simulink model "ComplianceSpeedgoat"  (R2025a)
settings: Solver=FixedStepAuto  StartTime=0.0  StopTime=inf  RelTol=1e-3
undefined symbols (not defined in the file or in its folder): HS, IO291
libraries: slrealtimeethercatlib x11, aru_toolbox x6, speedgoatlib_IO691 x1, speedgoatlib_IO291 x1
settings Model: SimulationMode=external  ExtModeEnableFloating=off  Creator=Blue Fifth  LastModifiedBy=user
settings SolverCC: ConcurrentTasks=on  PositivePriorityOrder=on  AutoInsertRateTranBlk=on
settings OptimizationCC: BlockReduction=off  OptimizeBlockIOStorage=off
settings DebuggingCC: TasksWithSamePriorityMsg=none
settings HardwareCC: ProdBitPerLong=64.0  ProdLongLongMode=on  ProdHWDeviceType=Intel->x86-64 (Linux 64)
settings RTWCC: SystemTargetFile=speedgoat.tlc  TemplateMakefile=slrealtime_default_tmf  Toolchain=Simulink Real-Time Toolchain  BuildConfiguration=Faster Runs  CodeExecutionProfiling=on  TargetLang=C++  GPUComputeCapability=3.5  Description=Speedgoat Real-Time Target Machine
settings SimulinkRealTimeTargetCC: SLRTFileLogMaxRuns=1.0  ExtModeMaxTrigDuration=10.0  ExtModeStaticAllocSize=1000000.0  ExtModeTransport=0.0  MultiwordLength=2048.0  DynamicStringBufferSize=256.0  PreserveMATLABNamespacesInGeneratedCode=on  SubcomponentCodeInterfacePackaging=Reusable function  InstructionSetFMA=off  LogToMDFFile=off

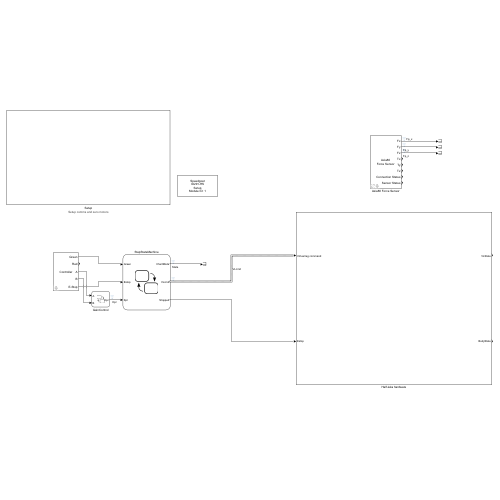
[thumbnail: Simulink's stored preview of the top-level diagram]
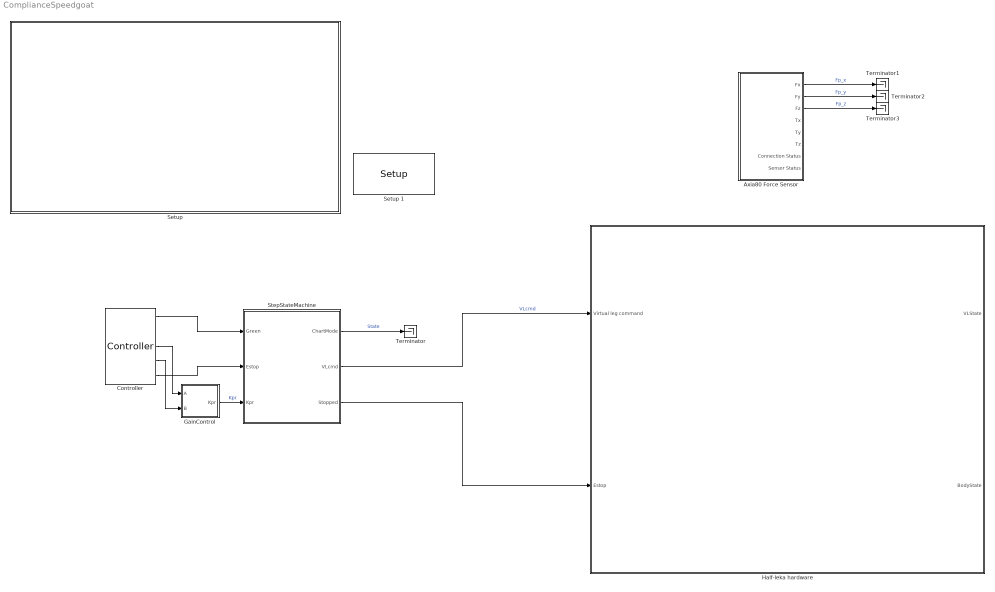
== system ComplianceSpeedgoat ==
  Axia80 Force Sensor : Subsystem  AncestorBlock=aru_toolbox/Axia80 Force Sensor  mask(Axia80 Force Sensor){resetBias=on, calibrationRangeParam=Range 0 (500N Fxy, 900N Fz, 20Nm Txyz), calibrationRangeTable={'0','500N','900N','20Nm'; '1','200N','360N','8Nm'}, sampleRateParam=975Hz, filterParam=No filtering (200Hz @ 0.5kHz, 350Hz @ 1kHz, 500Hz @ 2kHz, 1000Hz @ 4kHz), filterCutoffTable={'0','200','350','500','1000'; '1','58','115','235','460'; '2','22','45','90','180'; '3','10','21','43','84'; '4','5','10','20','40'; '5','2.5','5','10','20'; '6','1.3','3','5','10'; '7','0.6','1.2','2.4','4.7'; '8','0.3','0.7','1.4','2.7';}}
      mask prompts: resetBias "Reset Bias"; calibrationRangeParam "Calibration Range:"; calibrationRangeTable "Axia80-M20 Calibration Ranges"; sampleRateParam "Sample Rate:"; filterParam "Filter:"; filterCutoffTable "Filter -3dB Cutoff Frequency (in Hz) based on Sample Rate"
      mask help: <a href="matlab: web('https://www.ati-ia.com/app_content/documents/9610-05-EtherCAT%20Axia.pdf','-browser');">Axia80 EtherCAT Manual</a>
      mask TypeOptions calibrationRangeParam: Range 0 (500N Fxy, 900N Fz, 20Nm Txyz) | Range 1 (200N Fxy, 360N Fz, 8Nm Txyz)
      mask TypeOptions sampleRateParam: 487Hz | 975Hz | 1990Hz | 3900Hz
      mask TypeOptions filterParam: No filtering (200Hz @ 0.5kHz, 350Hz @ 1kHz, 500Hz @ 2kHz, 1000Hz @ 4kHz) | Filter 1 (58Hz @ 0.5kHz, 115Hz @ 1kHz, 235Hz @ 2kHz, 460Hz @ 4kHz) | Filter 2  (22Hz @ 0.5kHz, 45Hz @ 1kHz, 90Hz @ 2kHz, 180Hz @ 4kHz) | Filter 3  (10Hz @ 0.5kHz, 21Hz @ 1kHz, 43Hz @ 2kHz, 84Hz @ 4kHz) | Filter 4 (5Hz @ 0.5kHz, 10Hz @ 1kHz, 20Hz @ 2kHz, 40Hz @ 4kHz) | Filter 5 (2.5Hz @ 0.5kHz, 5Hz @ 1kHz, 10Hz @ 2kHz, 20Hz @ 4kHz) | Filter 6  (1.3Hz @ 0.5kHz, 3Hz @ 1kHz, 5Hz @ 2kHz, 10Hz @ 4kHz) | Filter 7  (0.6Hz @ 0.5kHz, 1.2Hz @ 1kHz, 2.4Hz @ 2kHz, 4.7Hz @ 4kHz) | Filter 8  (0.3Hz @ 0.5kHz, 0.7Hz @ 1kHz, 1.4Hz @ 2kHz, 2.7Hz @ 4kHz)
      mask Display:
      | disp('Axia80\nForce Sensor');
      | port_label('output',1,'Fx');
      | port_label('output',2,'Fy');
      | port_label('output',3,'Fz');
      | port_label('output',4,'Tx');
      | port_label('output',5,'Ty');
      | port_label('output',6,'Tz');
      | port_label('output',7,'Connection Status');
      | port_label('output',8,'Sensor Status');
  Controller : aru_toolbox/Controller
      settings: SourceProductName=ARU Toolbox
  GainControl : Stateflow chart  TreatAsAtomicUnit=on
  Half-leka hardware : Subsystem
  Setup : Subsystem
      settings: AttributesFormatString=Setup comms and zero motors
  Setup 1 : speedgoatlib_IO291/Setup   parInternalModuleId=1  parPciSlot=-1  parModuleId=1  parModuleType=IO291-HS  parTtlDoChannels=[]  parTtlDoInitValues=1  parTtlDoReset=1  parTtlDiChannels=[1 2 3 4 5]  parIsolDiChannels=[]  parFetDoChannels=[1 2 3 4 5 6]  parFetDoInitValues=0  parFetDoReset=1
      settings: SourceProductName=IO291
  StepStateMachine : Stateflow chart  TreatAsAtomicUnit=on
  Terminator{,1..3} (4 alike) : Terminator
  wires:
  StepStateMachine/2(VLcmd) -> Half-leka hardware/1(Virtual leg command)  "VLcmd"
  Controller/1 -> StepStateMachine/1(Green)
  StepStateMachine/1(ChartMode) -> Terminator/1  "State"
  Controller/5 -> StepStateMachine/2(Estop)
  StepStateMachine/3(Stopped) -> Half-leka hardware/2(Estop)
  Axia80 Force Sensor/1(Fx) -> Terminator1/1  "Fp_x"
  Axia80 Force Sensor/2(Fy) -> Terminator2/1  "Fp_y"
  Axia80 Force Sensor/3(Fz) -> Terminator3/1  "Fp_z"
  GainControl/1(Kpr) -> StepStateMachine/3(Kpr)  "Kpr"
  Controller/3 -> GainControl/1(A)
  Controller/4 -> GainControl/2(B)

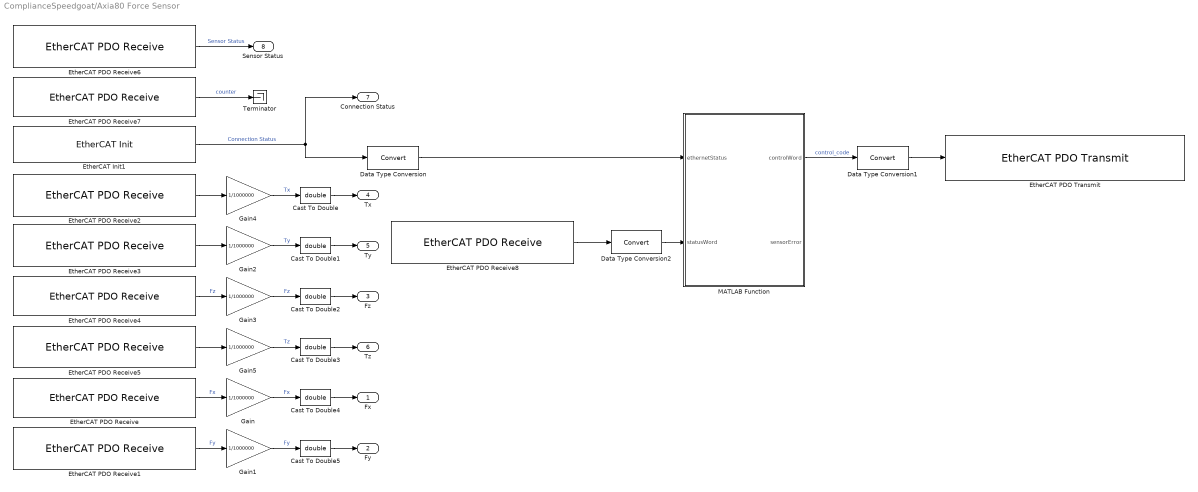
== system ComplianceSpeedgoat/Axia80 Force Sensor ==
  Cast To Double{,1..5} (6 alike) : DataTypeConversion  OutDataTypeStr=double  SaturateOnIntegerOverflow=off  RndMeth=Floor
  Data Type Conversion : DataTypeConversion  SaturateOnIntegerOverflow=off  RndMeth=Floor
  Data Type Conversion1 : DataTypeConversion  SaturateOnIntegerOverflow=off  RndMeth=Floor
  Data Type Conversion2 : DataTypeConversion  SaturateOnIntegerOverflow=off  RndMeth=Floor
  EtherCAT Init1 : slrealtimeethercatlib/EtherCAT Init  Priority=0  config_file=C:\Users\user\Documents\MATLAB\simulink-toolbox\Extras\axia80_ethercat_config.xml  device_id=0  portnum=1  initstate=2  dctuning=0  enaDebug=0  logFile='c:\dbglog.txt'  sample_time=0.001000  DCMode=0
  EtherCAT PDO Receive : slrealtimeethercatlib/EtherCAT PDO Receive  Priority=2  sig_name=Term 1 (ATI Axia F/T Sensor).Reading Data.Fx  sig_offset=312  sig_type=int32  type_size=32  sig_dim=1  device_id=0  sample_time=0.001000
  EtherCAT PDO Receive1 : slrealtimeethercatlib/EtherCAT PDO Receive  Priority=2  sig_name=Term 1 (ATI Axia F/T Sensor).Reading Data.Fy  sig_offset=344  sig_type=int32  type_size=32  sig_dim=1  device_id=0  sample_time=0.001000
  EtherCAT PDO Receive2 : slrealtimeethercatlib/EtherCAT PDO Receive  Priority=2  sig_name=Term 1 (ATI Axia F/T Sensor).Reading Data.Tx  sig_offset=408  sig_type=int32  type_size=32  sig_dim=1  device_id=0  sample_time=0.001000
  EtherCAT PDO Receive3 : slrealtimeethercatlib/EtherCAT PDO Receive  Priority=2  sig_name=Term 1 (ATI Axia F/T Sensor).Reading Data.Ty  sig_offset=440  sig_type=int32  type_size=32  sig_dim=1  device_id=0  sample_time=0.001000
  EtherCAT PDO Receive4 : slrealtimeethercatlib/EtherCAT PDO Receive  Priority=2  sig_name=Term 1 (ATI Axia F/T Sensor).Reading Data.Fz  sig_offset=376  sig_type=int32  type_size=32  sig_dim=1  device_id=0  sample_time=0.001000
  EtherCAT PDO Receive5 : slrealtimeethercatlib/EtherCAT PDO Receive  Priority=2  sig_name=Term 1 (ATI Axia F/T Sensor).Reading Data.Tz  sig_offset=472  sig_type=int32  type_size=32  sig_dim=1  device_id=0  sample_time=0.001000
  EtherCAT PDO Receive6 : slrealtimeethercatlib/EtherCAT PDO Receive  Priority=2  sig_name=Term 1 (ATI Axia F/T Sensor).Reading Data.Status Code  sig_offset=504  sig_type=uint32  type_size=32  sig_dim=1  device_id=0  sample_time=0.001000
  EtherCAT PDO Receive7 : slrealtimeethercatlib/EtherCAT PDO Receive  Priority=2  sig_name=Term 1 (ATI Axia F/T Sensor).Reading Data.Sample Counter  sig_offset=536  sig_type=uint32  type_size=32  sig_dim=1  device_id=0  sample_time=0.001000
  EtherCAT PDO Receive8 : slrealtimeethercatlib/EtherCAT PDO Receive  Priority=2  sig_name=Term 1 (ATI Axia F/T Sensor).Reading Data.Status Code  sig_offset=504  sig_type=uint32  type_size=32  sig_dim=1  device_id=0  sample_time=0.001000
  EtherCAT PDO Transmit : slrealtimeethercatlib/EtherCAT PDO Transmit  Priority=3  sig_name=Term 1 (ATI Axia F/T Sensor).Control Codes.Control 1  sig_offset=312  sig_type=uint32  type_size=32  sig_dim=1  device_id=0  sample_time=0.001000
  Gain{,1..5} (6 alike) : Gain  Gain=1/1000000
  MATLAB Function : MATLAB Function  TreatAsAtomicUnit=on
  Terminator : Terminator
  Fx : Outport
  Fy : Outport  Port=2
  Fz : Outport  Port=3
  Tx : Outport  Port=4
  Ty : Outport  Port=5
  Tz : Outport  Port=6
  Connection Status : Outport  Port=7
  Sensor Status : Outport  Port=8
  wires:
  Cast To Double5/1 -> Fy/1
  Cast To Double4/1 -> Fx/1
  Cast To Double3/1 -> Tz/1
  Cast To Double2/1 -> Fz/1
  Cast To Double1/1 -> Ty/1
  Cast To Double/1 -> Tx/1
  Data Type Conversion2/1 -> MATLAB Function/2(statusWord)
  EtherCAT PDO Receive8/1 -> Data Type Conversion2/1
  EtherCAT PDO Receive4/1 -> Gain3/1  "Fz"
  Gain3/1 -> Cast To Double2/1  "Fz"
  EtherCAT PDO Receive5/1 -> Gain5/1
  EtherCAT PDO Receive7/1 -> Terminator/1  "counter"
  EtherCAT PDO Receive6/1 -> Sensor Status/1  "Sensor Status"
  Gain/1 -> Cast To Double4/1  "Fx"
  EtherCAT PDO Receive/1 -> Gain/1  "Fx"
  Gain5/1 -> Cast To Double3/1  "Tz"
  Gain1/1 -> Cast To Double5/1  "Fy"
  EtherCAT PDO Receive3/1 -> Gain2/1
  Data Type Conversion1/1 -> EtherCAT PDO Transmit/1
  Gain2/1 -> Cast To Double1/1  "Ty"
  EtherCAT Init1/1 -> Data Type Conversion/1, Connection Status/1  "Connection Status"
  EtherCAT PDO Receive1/1 -> Gain1/1  "Fy"
  Data Type Conversion/1 -> MATLAB Function/1(ethernetStatus)
  Gain4/1 -> Cast To Double/1  "Tx"
  EtherCAT PDO Receive2/1 -> Gain4/1
  MATLAB Function/1(controlWord) -> Data Type Conversion1/1  "control_code"

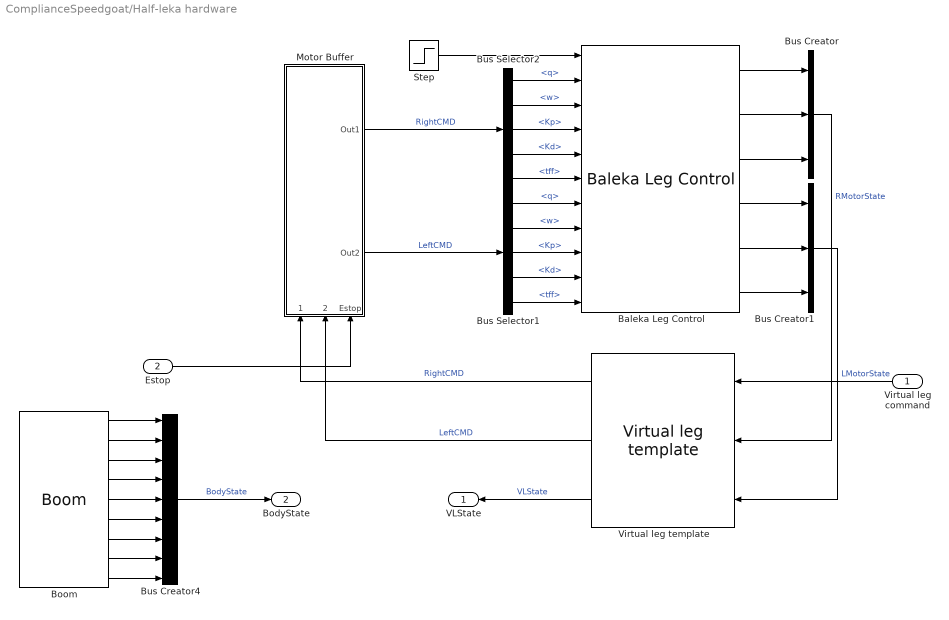
== system ComplianceSpeedgoat/Half-leka hardware ==
  Virtual leg command : Inport
  Estop : Inport  Port=2
  Baleka Leg Control : aru_toolbox/Baleka 2.5/Baleka Leg Control  CAN_ID_L=6  CAN_ID_R=5  channel=2  Comm_freq=1000  enableOffsets=on  KtuneL=1.1986  KtuneR=1.2249
      link override CAN Read/CAN Read Command: canType=CAN (HS)
      settings: SourceProductName=ARU Toolbox
  Boom : aru_toolbox/Boom  ts=0.001
      settings: SourceProductName=ARU Toolbox
  Bus Creator : BusCreator  Inputs=3  OutDataTypeStr=Bus: MotorState  NonVirtualBus=on
      settings: InheritFromInputs=off
  Bus Creator1 : BusCreator  Inputs=3  OutDataTypeStr=Bus: MotorState  NonVirtualBus=on
      settings: InheritFromInputs=off
  Bus Creator4 : BusCreator  Inputs=9  OutDataTypeStr=Bus: BodyState  NonVirtualBus=on
  Bus Selector1 : BusSelector  OutputSignals=q,w,Kp,Kd,tff
  Bus Selector2 : BusSelector  OutputSignals=q,w,Kp,Kd,tff
  Motor Buffer : Subsystem
      settings: AttributesFormatString=Lets the motors read for 1s before applying any commands (to remove initial spikes interfering with control)  PortSchema="{\"entries\":[{\"content\":{\"sides\":[{\"content\":{},\"type\":\"ConnectorPlacement.EquallySpacedRectSide\",\"uuid\":\"27edc325-da8c-4b2d-b123-f87d1cc3e5bc\"},{\"content\":{\"connectorIds\":[\"Out1\",\"Out2\"],\"side\":\"RIGHT\"},\"type\":\"ConnectorPlacement.EquallySpacedRectSide\",\"uuid\":\"f90c51b7-dac4-4b26-9893-9f73a92cc20e\"},{\"content\":{\"side\":\"TOP\"},\"type\":\"ConnectorPlacement.EquallySpacedRectSide\",\"uuid\":\"2a4858a0-4733-4976-9a98-0a846159363f\"},{\"content\":{\"connectorIds\":[\"In1\",\"In2\",\"In3\"],\"side\":\"BOTTOM\"},\"type\":\"ConnectorPlacement.EquallySpacedRectSide\",\"uuid\":\"7b6afc87-1c19-49ec-a782-e05d81e1c271\"}]},\"type\":\"ConnectorPlacement.EquallySpacedConnector\",\"uuid\":\"20e3ed70-affb-44e3-a10c-c85a1a7632d2\"}],\"packageUris\":[\"http://schema.mathworks.com/mf0/Connector/R2020b\"],\"version\":\"1.0\"}"
  Step : Step  Time=4  SampleTime=0
  Virtual leg template : aru_toolbox/Baleka 2.5/Virtual leg template  mx_tune=0.5543  cx_tune=-1.076  my_tune=0.6663  cy_tune=-10.6614
      settings: SourceProductName=ARU Toolbox
  VLState : Outport
  BodyState : Outport  Port=2
  wires:
  Bus Creator/1 -> Virtual leg template/2  "RMotorState"
  Baleka Leg Control/6 -> Bus Creator1/3
  Bus Selector2/4 -> Baleka Leg Control/5  "<Kd>"
  Baleka Leg Control/2 -> Bus Creator/2
  Bus Selector2/1 -> Baleka Leg Control/2  "<q>"
  Baleka Leg Control/1 -> Bus Creator/1
  Bus Creator1/1 -> Virtual leg template/3  "LMotorState"
  Step/1 -> Baleka Leg Control/1
  Baleka Leg Control/4 -> Bus Creator1/1
  Baleka Leg Control/3 -> Bus Creator/3
  Bus Selector2/5 -> Baleka Leg Control/6  "<tff>"
  Bus Selector2/3 -> Baleka Leg Control/4  "<Kp>"
  Bus Selector1/3 -> Baleka Leg Control/9  "<Kp>"
  Bus Selector1/2 -> Baleka Leg Control/8  "<w>"
  Baleka Leg Control/5 -> Bus Creator1/2
  Bus Selector2/2 -> Baleka Leg Control/3  "<w>"
  Bus Selector1/5 -> Baleka Leg Control/11  "<tff>"
  Bus Selector1/1 -> Baleka Leg Control/7  "<q>"
  Bus Selector1/4 -> Baleka Leg Control/10  "<Kd>"
  Virtual leg command/1 -> Virtual leg template/1
  Boom/2 -> Bus Creator4/2
  Boom/8 -> Bus Creator4/8
  Boom/1 -> Bus Creator4/1
  Bus Creator4/1 -> BodyState/1  "BodyState"
  Boom/3 -> Bus Creator4/3
  Boom/5 -> Bus Creator4/5
  Boom/6 -> Bus Creator4/6
  Boom/7 -> Bus Creator4/7
  Boom/4 -> Bus Creator4/4
  Virtual leg template/1 -> Motor Buffer/1(RightCMD)  "RightCMD"
  Virtual leg template/2 -> Motor Buffer/2(LeftCMD)  "LeftCMD"
  Motor Buffer/1(Out1) -> Bus Selector2/1  "RightCMD"
  Motor Buffer/2(Out2) -> Bus Selector1/1  "LeftCMD"
  Boom/9 -> Bus Creator4/9
  Virtual leg template/3 -> VLState/1  "VLState"
  Estop/1 -> Motor Buffer/3(Estop)

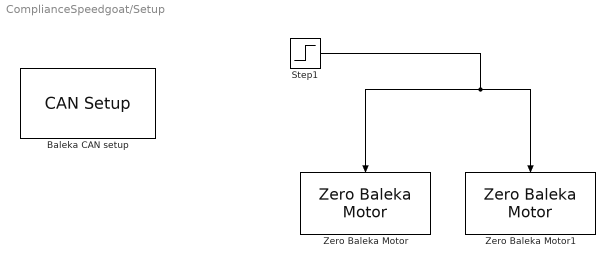
== system ComplianceSpeedgoat/Setup ==
  Baleka CAN setup : speedgoatlib_IO691/Legacy/CAN Setup   moduletype=IO691  id=1  pciSlot=-1  chn1=CAN (HS)  chn2=CAN (HS)  chn3=Disabled  chn4=Disabled  initStruct=[]  termStruct=[struct('Channel',1,'Protocol','CAN','BRS',0,'Type','Extended','Identifier',1,'Data',[255, 255, 255, 255, 255, 255, 255, 253],'Pause',0.001), struct('Channel',2,'Protocol','CAN','BRS',0,'Type','Standard','Identifier',2,'Data',[255, 255, 255, 255, 255, 255, 255, 253],'Pause',0.001)]  ArbitrationbdrChn1=1.0 MBaud  ArbitrationManbdrChn1=[2,8,31,8]  FdbdrChn1=1.0 MBaud  FdManbdrChn1=[2,8,31,8]  ArbitrationbdrChn2=1.0 MBaud  ArbitrationManbdrChn2=[2,8,31,8]  FdbdrChn2=1.0 MBaud  FdManbdrChn2=[2,8,31,8]  ArbitrationbdrChn3=1.0 MBaud  ArbitrationManbdrChn3=[2,8,31,8]  FdbdrChn3=5.0 MBaud  FdManbdrChn3=[2,2,5,2]  ArbitrationbdrChn4=1.0 MBaud  ArbitrationManbdrChn4=[2,8,31,8]  FdbdrChn4=5.0 MBaud  FdManbdrChn4=[2,2,5,2]  moduleInitValues=[691 1 -1 -1]
      settings: SourceProductName=IO691
  Step1 : Step  Time=0.3  SampleTime=0
  Zero Baleka Motor : aru_toolbox/Baleka 2.5/Zero Baleka Motor  CAN_ID=1  channel=1
      settings: SourceProductName=ARU Toolbox
  Zero Baleka Motor1 : aru_toolbox/Baleka 2.5/Zero Baleka Motor  CAN_ID=2  channel=1
      settings: SourceProductName=ARU Toolbox
  wires:
  Step1/1 -> Zero Baleka Motor1/Trigger, Zero Baleka Motor/Trigger

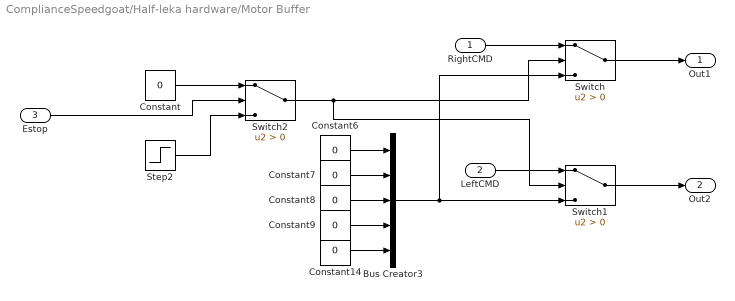
== system ComplianceSpeedgoat/Half-leka hardware/Motor Buffer ==
  RightCMD : Inport
  LeftCMD : Inport  Port=2
  Estop : Inport  Port=3
  Bus Creator3 : BusCreator  Inputs=5  OutDataTypeStr=Bus: MotorCmd  NonVirtualBus=on
      settings: InheritFromInputs=off
  Constant{,6..9,14} (6 alike) : Constant  Value=0
  Step2 : Step  Time=5  SampleTime=0
  Switch : Switch  Criteria=u2 > Threshold  SaturateOnIntegerOverflow=off  InputSameDT=off
  Switch1 : Switch  Criteria=u2 > Threshold  SaturateOnIntegerOverflow=off  InputSameDT=off
  Switch2 : Switch  Criteria=u2 > Threshold  SaturateOnIntegerOverflow=off  InputSameDT=off
  Out1 : Outport
  Out2 : Outport  Port=2
  wires:
  LeftCMD/1 -> Switch1/1
  Bus Creator3/1 -> Switch/3, Switch1/3
  Constant7/1 -> Bus Creator3/2
  Constant9/1 -> Bus Creator3/4
  Constant8/1 -> Bus Creator3/3
  Constant6/1 -> Bus Creator3/1
  Constant14/1 -> Bus Creator3/5
  Switch/1 -> Out1/1
  Switch1/1 -> Out2/1
  RightCMD/1 -> Switch/1
  Switch2/1 -> Switch1/2, Switch/2
  Step2/1 -> Switch2/3
  Constant/1 -> Switch2/1
  Estop/1 -> Switch2/2

== stateflow chart ComplianceSpeedgoat/GainControl ==
  state Starting_gain
    Kpr = 1000;
  state Gain2
    Kpr = 1250;
  state Gain3
    Kpr = 1500;
  state Gain4
    Kpr = 1750;
  state Gain5
    Kpr = 2000;
  (default) -> Starting_gain
  Gain2 -> Starting_gain [order 2] : [[B >0 & after(500, msec)]]
  Starting_gain -> Gain2 : [A >0 & after(500, msec)]
  Gain3 -> Gain2 [order 2] : [B >0 & after(500, msec)]
  Gain2 -> Gain3 [order 1] : [A >0 & after(500, msec)]
  Gain4 -> Gain3 [order 1] : [B >0 & after(500, msec)]
  Gain3 -> Gain4 [order 1] : [A >0 & after(500, msec)]
  Gain5 -> Gain4 : [B >0 & after(500, msec)]
  Gain4 -> Gain5 [order 2] : [A >0 & after(500, msec)]
  data: A input; B input; Kpr output

== matlab function ComplianceSpeedgoat/Axia80 Force Sensor/MATLAB Function ==
  data: ethernetStatus input; controlWord output; statusWord input; sensorError output; resetBias parameter; calibrationRangeParam parameter; sampleRateParam parameter; filterParam parameter
function [controlWord, sensorError] = fcn(ethernetStatus, statusWord, resetBias, calibrationRangeParam, sampleRateParam, filterParam)

% Control Words
% https://www.ati-ia.com/app_content/documents/9610-05-EtherCAT%20Axia.pdf
% page 41

filter = dec2bin(filterParam-1,4); % no filtering
calibrationRange = dec2bin(calibrationRangeParam-1,4); % 0:Fz=900N, 1:Fz=360N
sampleRate = dec2bin(sampleRateParam-1,4); % 0=487Hz, 1=975Hz, 2=1990Hz, 3=3900Hz
Reserved = dec2bin(0,1); % 1 bit reserved placeholder

offsetBias = dec2bin(1,1); % 1=set bias against current load
clearBias = dec2bin(0,1); % 0=leave bias unchanged
setBias = bin2dec([sampleRate, calibrationRange, filter, Reserved, clearBias, Reserved, offsetBias]);

offsetBias = dec2bin(0,1); % 0=use last set bias
clearBias = dec2bin(0,1); % 0=leave bias unchanged
normalOp = bin2dec([sampleRate, calibrationRange, filter, Reserved, clearBias, Reserved, offsetBias]);


persistent iterationNo
if(isempty(iterationNo))
    iterationNo = 0;
end

% FT Sensors
if (ethernetStatus(2)==8) % if ethernet has been enabled and in OP mode
    if iterationNo < 4
        if (resetBias == 1)
            controlWord = setBias; % Set bias
        else
            controlWord = normalOp;
        end
        iterationNo = iterationNo + 1;
    else
        controlWord = normalOp;
    end
    
    if (bitand(statusWord, 2147483648))
        sensorError = 1; % if there is an error
    else
        sensorError = 0;
    end
else
    controlWord = normalOp;
    sensorError = 0;
end

out = sampleRateParam;

== stateflow chart ComplianceSpeedgoat/StepStateMachine ==
  state EnableCompliance
    % Static values
    VLcmd.Tff = 0;
    VLcmd.dth_des =0;
    VLcmd.th_des = -pi/2;
    VLcmd.KPth = 350;
    VLcmd.KDth = 10;
    % Springy time
    VLcmd.r_des = 0.45;
    VLcmd.dr_des =0;
    VLcmd.KPr = Kpr;
    VLcmd.KDr =150;
    VLcmd.Fff =0;
  state StandUp
    Stopped = 0;
    % Static values
    VLcmd.Tff = 0;
    VLcmd.dth_des =0;
    VLcmd.th_des = -pi/2;
    VLcmd.KPth = 50;
    VLcmd.KDth = 5;
    % Gentle stand-up
    VLcmd.r_des = 0.30;
    VLcmd.dr_des =0;
    VLcmd.KPr = 600;
    VLcmd.KDr =50;
    VLcmd.Fff =0;
  state Further_up
    % Static values
    VLcmd.Tff = 0;
    VLcmd.dth_des =0;
    VLcmd.th_des = -pi/2;
    VLcmd.KPth = 50;
    VLcmd.KDth = 5;
    % Gentle stand-up
    VLcmd.r_des = 0.45;
    VLcmd.dr_des =0;
    VLcmd.KPr = 600;
    VLcmd.KDr =50;
    VLcmd.Fff =0;
  state Estop
    % Static values
    VLcmd.Tff = 0;
    VLcmd.dth_des =0;
    VLcmd.th_des = 0;
    VLcmd.KPth = 0;
    VLcmd.KDth = 0;
    VLcmd.r_des = 0;
    VLcmd.dr_des =0;
    VLcmd.KPr = 0;
    VLcmd.KDr =0;
    VLcmd.Fff =0;
    Stopped = 1;
  (default) -> StandUp
  EnableCompliance -> StandUp [order 1] : [Green>0 & after(500, msec)]
  EnableCompliance -> Estop [order 2] : [Estop>0]
  Further_up -> EnableCompliance [order 1] : [after(1, sec)]
  StandUp -> Estop [order 2] : [Estop>0]
  StandUp -> Further_up [order 1] : [Green >0 & after(500, msec)]
  Further_up -> Estop [order 2] : [Estop>0]
  data: ChartMode output Enum: ChartModeType; VLcmd output Bus: VLcmd; Green input; Estop input; Stopped output; Kpr input double
